simulink model "eg1"  (R2021a)
settings: Solver=VariableStepAuto  StartTime=0.0  StopTime=10  FixedStep=0.01  RelTol=1e-6
settings Model: Creator=lilic  LastModifiedBy=Jieming

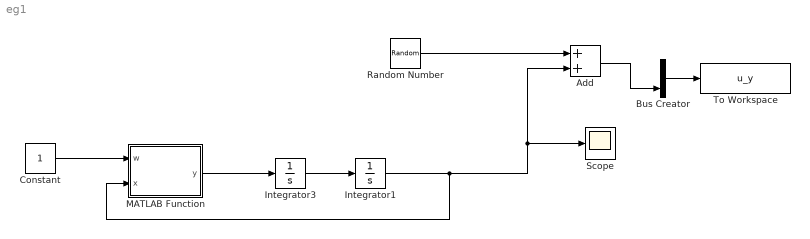
== system eg1 ==
  Add : Sum
  Bus Creator : BusCreator  Inputs=2
  Constant : Constant
  Integrator1 : Integrator  InitialCondition=0.0001
  Integrator3 : Integrator  InitialCondition=0.9998
  MATLAB Function : MATLAB Function  TreatAsAtomicUnit=on
  Random Number : RandomNumber  Variance=0.0001
  Scope : Scope
  To Workspace : ToWorkspace  VariableName=u_y  SaveFormat=Timeseries  SampleTime=0.01
  wires:
  Bus Creator/1 -> To Workspace/1
  Constant/1 -> MATLAB Function/1(w)
  Random Number/1 -> Add/1
  Add/1 -> Bus Creator/2
  MATLAB Function/1(y) -> Integrator3/1
  Integrator3/1 -> Integrator1/1
  Integrator1/1 -> MATLAB Function/2(x), Scope/1, Add/2

== matlab function eg1/MATLAB Function ==
  data: w input; y output; x input
function y = fcn(w,x)
y = -w^2*x
